simulink model "mod3_2plus1SMASH"  (Simulink 8.1)
settings: Solver=FixedStepDiscrete  StartTime=0.0  StopTime=80e-3  RelTol=1e-3
undefined symbols (not defined in the file): Fs, modctrl
libraries: dspsigops x3, dspsrcs4 x2
settings Model: MinMaxOverflowLogging=ForceOff  Creator=amyles  LastModifiedBy=amyles
settings DataIOCC: LimitDataPoints=off  MaxDataPoints=50000  SaveOutput=off  SaveTime=off
settings OptimizationCC: InlineParams=on
settings DebuggingCC: StrictBusMsg=Warning
settings ModelReferenceCC: ModelReferenceNumInstancesAllowed=Single

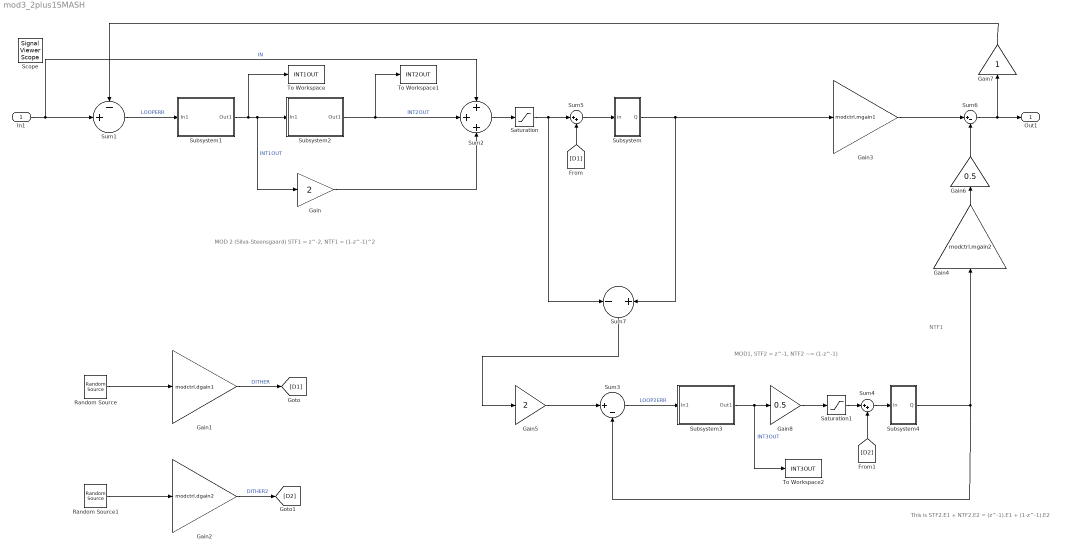
== system mod3_2plus1SMASH ==
  note: MOD 2 (Silva-Steensgaard)
      | STF1 = z^-2, NTF1 = (1-z^-1)^2
  note: MOD1, STF2 = z^-1, NTF2 ~= (1-z^-1)
  note: This is STF2.E1 + NTF2.E2
      | = (z^-1).E1 + (1-z^-1).E2
  note: NTF1
  In1 : Inport
  Gain : Gain  Gain=2
  Gain1 : Gain  Gain=modctrl.dgain1
      settings: AttributesFormatString=Dither level adjust
  Gain2 : Gain  Gain=modctrl.dgain2
      settings: AttributesFormatString=Dither level adjust
  Gain3 : Gain  Gain=modctrl.mgain1
  Gain4 : Gain  Gain=modctrl.mgain2
  Gain5 : Gain  Gain=2
      settings: AttributesFormatString=Option to scale input\nfor saturation control...
  Gain6 : Gain  Gain=0.5
      settings: AttributesFormatString=Option to un-scale input\npost saturation control...
  Gain7 : Gain
      settings: AttributesFormatString=Option to un-scale input\npost saturation control...
  Gain8 : Gain  Gain=0.5
      settings: AttributesFormatString=Option to scale input\nfor saturation control...
  Random Source : dspsrcs4/Random Source  SrcType=Uniform  NormMethod=Ziggurat  CltLength=12  MinVal=-1  MaxVal=1  MeanVal=0  VarVal=1  RepMode=Not repeatable  rawSeed=1  IsInherit=off  SampMode=Discrete  SampTime=1/Fs  SampFrame=1  DataType=Double  OutComplex=Real
      settings: AttributesFormatString=Dither source
  Random Source1 : dspsrcs4/Random Source  SrcType=Uniform  NormMethod=Ziggurat  CltLength=12  MinVal=-1  MaxVal=1  MeanVal=0  VarVal=1  RepMode=Not repeatable  rawSeed=1  IsInherit=off  SampMode=Discrete  SampTime=1/Fs  SampFrame=1  DataType=Double  OutComplex=Real
      settings: AttributesFormatString=Dither source
  Saturation : Saturate  UpperLimit=modctrl.qsatin1  LowerLimit=-(modctrl.qsatin1)
  Saturation1 : Saturate  UpperLimit=modctrl.qsatin2  LowerLimit=-(modctrl.qsatin2)
  Subsystem : Subsystem
      settings: AttributesFormatString=2-bit quantiser
  Subsystem1 : Subsystem
      settings: AttributesFormatString=Leaky delaying int
  Subsystem2 : Subsystem
      settings: AttributesFormatString=Leaky delaying int
  Subsystem3 : Subsystem
      settings: AttributesFormatString=Leaky delaying int
  Subsystem4 : Subsystem
      settings: AttributesFormatString=2-bit quantiser
  Sum1 : Sum  Inputs=-+|
      settings: AttributesFormatString=Modulator input\nloop servo error (input - fbk)
  Sum2 : Sum  Inputs=+++
  Sum3 : Sum  Inputs=|+-
      settings: AttributesFormatString=Modulator input\nloop servo error (input - fbk)
  Sum4 : Sum  Inputs=|++
  Sum5 : Sum  Inputs=|++
  Sum6 : Sum  Inputs=|+-
  Sum7 : Sum  Inputs=-|+
  To Workspace : ToWorkspace  VariableName=INT1OUT  SampleTime=-1
  To Workspace1 : ToWorkspace  VariableName=INT2OUT  SampleTime=-1
  To Workspace2 : ToWorkspace  VariableName=INT3OUT  SampleTime=-1
  Out1 : Outport
  Scope : SignalViewerScope  IOType=viewer  NumInputPorts=3  ZoomMode=yonly  RefreshTime=0.035000
      settings: YMin=-5~-5~-15  YMax=5~5~15
  wires:
  Sum1/1 -> Subsystem1/1(In1)  "LOOPERR"
  In1/1 -> Sum2/1, Sum1/2  "IN"
  Random Source/1 -> Gain1/1
  Gain/1 -> Sum2/3
  Sum5/1 -> Subsystem/1(in)
  Sum3/1 -> Subsystem3/1(In1)  "LOOP2ERR"
  Subsystem1/1(Out1) -> Subsystem2/1(In1), Gain/1, To Workspace/1  "INT1OUT"
  Sum2/1 -> Saturation/1
  Subsystem3/1(Out1) -> Gain8/1, To Workspace2/1  "INT3OUT"
  Sum4/1 -> Subsystem4/1(in)
  Subsystem4/1(Q) -> Sum3/2, Gain4/1
  Random Source1/1 -> Gain2/1
  Gain3/1 -> Sum6/1
  Gain4/1 -> Gain6/1
  Sum6/1 -> Out1/1, Gain7/1
  Gain5/1 -> Sum3/1
  Gain6/1 -> Sum6/2
  Subsystem/1(Q) -> Sum7/2, Gain3/1
  Gain1/1 -> [D1]  "DITHER"
  Gain2/1 -> [D2]  "DITHER2"
  [D1] -> Sum5/2
  [D2] -> Sum4/2
  Saturation/1 -> Sum5/1, Sum7/1
  Saturation1/1 -> Sum4/1
  Sum7/1 -> Gain5/1
  Subsystem2/1(Out1) -> Sum2/2, To Workspace1/1  "INT2OUT"
  Gain7/1 -> Sum1/1
  Gain8/1 -> Saturation1/1

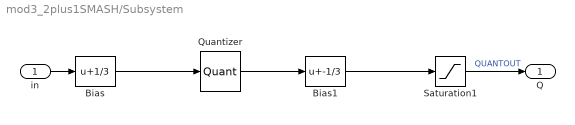
== system mod3_2plus1SMASH/Subsystem ==
  in : Inport
  Bias : Bias  Bias=1/3
      settings: AttributesFormatString=Need offset to give\nMID-RISE quantiser
  Bias1 : Bias  Bias=-1/3
  Quantizer : Quantizer  QuantizationInterval=2/3  LinearizeAsGain=off
  Saturation1 : Saturate  UpperLimit=1  LowerLimit=-1
      settings: AttributesFormatString=Limit quantiser\noutput to +/-1
  Q : Outport
  wires:
  Bias/1 -> Quantizer/1
  Quantizer/1 -> Bias1/1
  Bias1/1 -> Saturation1/1
  in/1 -> Bias/1
  Saturation1/1 -> Q/1  "QUANTOUT"

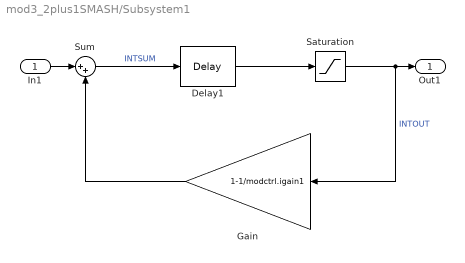
== system mod3_2plus1SMASH/Subsystem1 ==
  In1 : Inport
  Delay1 : dspsigops/Delay  dly_unit=Samples  delay=1  ic_detail=off  dif_ic_for_ch=off  dif_ic_for_dly=off  ic=0  reset_popup=None
  Gain : Gain  Gain=1-1/modctrl.igain1
      settings: AttributesFormatString=Integrator leakage
  Saturation : Saturate  UpperLimit=modctrl.isat1  LowerLimit=-(modctrl.isat1)
  Sum : Sum  Inputs=|++
      settings: AttributesFormatString=Integrator summer
  Out1 : Outport
  wires:
  Sum/1 -> Delay1/1  "INTSUM"
  Gain/1 -> Sum/2
  Saturation/1 -> Gain/1, Out1/1  "INTOUT"
  Delay1/1 -> Saturation/1
  In1/1 -> Sum/1

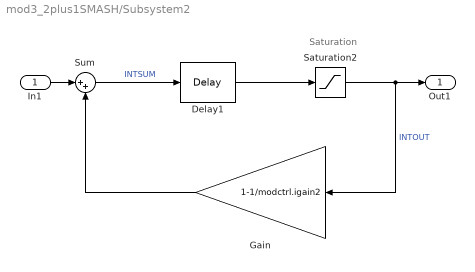
== system mod3_2plus1SMASH/Subsystem2 ==
  note: Saturation
  In1 : Inport
  Delay1 : dspsigops/Delay  dly_unit=Samples  delay=1  ic_detail=off  dif_ic_for_ch=off  dif_ic_for_dly=off  ic=0  reset_popup=None
  Gain : Gain  Gain=1-1/modctrl.igain2
      settings: AttributesFormatString=Integrator leakage
  Saturation2 : Saturate  UpperLimit=modctrl.isat2  LowerLimit=-(modctrl.isat2)
  Sum : Sum  Inputs=|++
      settings: AttributesFormatString=Integrator summer
  Out1 : Outport
  wires:
  In1/1 -> Sum/1
  Delay1/1 -> Saturation2/1
  Saturation2/1 -> Out1/1, Gain/1  "INTOUT"
  Gain/1 -> Sum/2
  Sum/1 -> Delay1/1  "INTSUM"

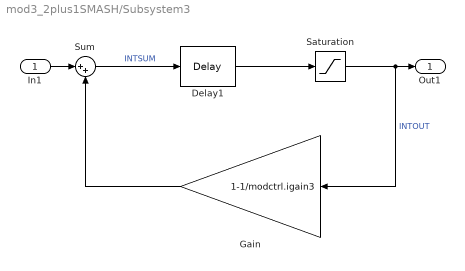
== system mod3_2plus1SMASH/Subsystem3 ==
  In1 : Inport
  Delay1 : dspsigops/Delay  dly_unit=Samples  delay=1  ic_detail=off  dif_ic_for_ch=off  dif_ic_for_dly=off  ic=0  reset_popup=None
  Gain : Gain  Gain=1-1/modctrl.igain3
      settings: AttributesFormatString=Integrator leakage
  Saturation : Saturate  UpperLimit=modctrl.isat3  LowerLimit=-(modctrl.isat3)
  Sum : Sum  Inputs=|++
      settings: AttributesFormatString=Integrator summer
  Out1 : Outport
  wires:
  In1/1 -> Sum/1
  Delay1/1 -> Saturation/1
  Saturation/1 -> Out1/1, Gain/1  "INTOUT"
  Gain/1 -> Sum/2
  Sum/1 -> Delay1/1  "INTSUM"

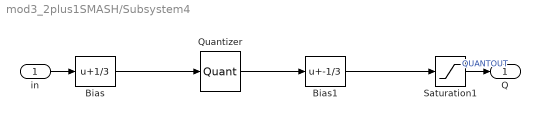
== system mod3_2plus1SMASH/Subsystem4 ==
  in : Inport
  Bias : Bias  Bias=1/3
      settings: AttributesFormatString=Need offset to give\nMID-RISE quantiser
  Bias1 : Bias  Bias=-1/3
  Quantizer : Quantizer  QuantizationInterval=2/3  LinearizeAsGain=off
  Saturation1 : Saturate  UpperLimit=1  LowerLimit=-1
      settings: AttributesFormatString=Limit quantiser\noutput to +/-1
  Q : Outport
  wires:
  Saturation1/1 -> Q/1  "QUANTOUT"
  in/1 -> Bias/1
  Bias1/1 -> Saturation1/1
  Quantizer/1 -> Bias1/1
  Bias/1 -> Quantizer/1
